simulink model "ExampleVariousBlocks"  (Simulink 9.2)
settings: Solver=FixedStepDiscrete  StartTime=0.0  StopTime=inf  FixedStep=0.001  RelTol=1e-3  EnableMultiTasking=on
InitFcn:
  | RFPRO_TIMESTEP = 1/1000;
  | 
  | % From c-code model
  | gCGHeight = 0.3545;            % height of the car body reference point above the ground
  | gLeftWheelBase = 3.105;        % distance between left front and rear axles
  | gRightWheelBase = 3.105;       % distance between right front and rear axles
  | gFrontTrack = 1.418;           % distance between front left and right wheels
  | gRearTrack = 1.412;            % distance between rear left and right wheels
  | gFrontWheelRadius = 0.32;
  | gRearWheelRadius = 0.33;
  | 
  | CG_OFFSET_FROM_NOSE = [-gLeftWheelBase/2, 0, gCGHeight];
libraries: rFproPhysicsLib x7, simulink x1
settings Model: Creator=enewton  LastModifiedBy=SeanKavanagh  ParamWorkspaceSource=ReferencedWorkspace  TunableVars=LOCAL_PORT_RECV,REMOTE_PORT_RECV,gCGHeight,gFrontTrack,gFrontWheelRadius,gLeftWheelBase,gRearTrack,gRearWheelRadius,gRightWheelBase  TunableVarsStorageClass=Auto,Auto,Auto,Auto,Auto,Auto,Auto,Auto,Auto  TunableVarsTypeQualifier=,,,,,,,,
settings DataIOCC: SaveOutput=off  SignalLogging=off  DSMLogging=off  SaveTime=off
settings OptimizationCC: BlockReduction=off  ConditionallyExecuteInputs=off  OptimizeBlockIOStorage=off  BufferReuse=off  GlobalBufferReuse=off  ExpressionFolding=off  ExpressionDepthLimit=2147483647  LocalBlockOutputs=off  OptimizeDataStoreBuffers=off  BusAssignmentInplaceUpdate=off
settings DebuggingCC: SolverPrmCheckMsg=warning
settings RTWCC: SystemTargetFile=rfpro.tlc  MakeCommand="make_rtw OPTS=\"-DRUN_PHYSICS\""  TemplateMakefile=rfpro.tmf  Description=rFpro Target (Run Physics)  TargetLang=C++
settings STFCustomTargetCC: ModelReferenceCompliant=off  GeneratePreprocessorConditionals=Disable all  CombineOutputUpdateFcns=on  MatFileLogging=on  CPPClassGenCompliant=on  GRTInterface=off  SystemTargetFile=rfpro.tlc
settings GRTTargetCC: ModelReferenceCompliant=off  ParMdlRefBuildCompliant=off  CompOptLevelCompliant=off  ConcurrentExecutionCompliant=off  CombineOutputUpdateFcns=on  GRTInterface=off  UseToolchainInfoCompliant=off

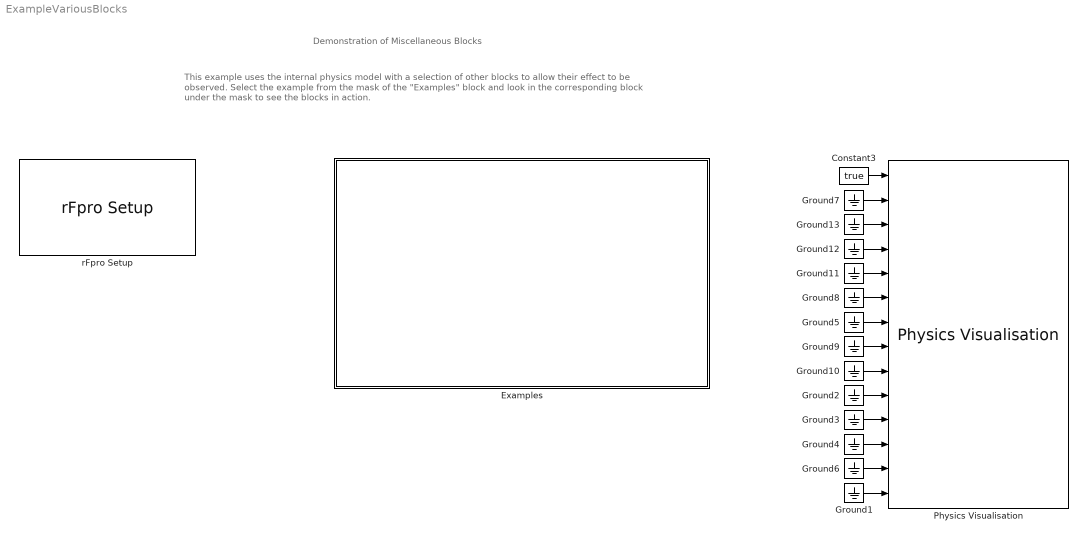
== system ExampleVariousBlocks ==
  note: This example uses the internal physics model with a selection of other blocks to allow their effect to be observed.
      | Select the example from the mask of the "Examples" block and look in the corresponding block under the mask to
      | see the blocks in action.
  note: Demonstration of Miscellaneous Blocks
  Constant3 : Constant  Value=true
  Examples : Subsystem  Variant=on  mask(rFpro Examples){activeExample=Send Command}
      mask prompts: activeExample "Active Example"
      mask help: Select the example you wish to use from the drop down box, and look in the subsystems to see the blocks in use.
      mask init:
      | assignin('base', 'rFpro_VariousBlocksExample', activeExample);
      | 
      | assignin('base', 'rFpro_VariousBlocksCmd', Simulink.Variant('rFpro_VariousBlocksExample == 1'));
      | assignin('base', 'rFpro_VariousBlocksFMOD', Simulink.Variant('rFpro_VariousBlocksExample == 2'));
      | assignin('base', 'rFpro_VariousBlocksTelem', Simulink.Variant('rFpro_VariousBlocksExample == 3'));
      | assignin('base', 'rFpro_VariousBlocksProx', Simulink.Variant('rFpro_VariousBlocksExample == 4'));
      | assignin('base', 'rFpro_VariousBlocksHead', Simulink.Variant('rFpro_VariousBlocksExample == 5'));
      mask TypeOptions activeExample: Send Command | FMOD Sound | Telemetry | Object Proximity | Head Tracking
      mask Display:
      | disp(['Current Example:\n\n' get_param(gcb, 'activeExample')])
      | if activeExample < 4
      |     text(0.2, 0.2, 'Note: external settings required. See under mask.')
      | end
  Ground{1..13} (13 alike) : Ground
  Physics Visualisation : rFproPhysicsLib/Physics Visualisation  PAR_SKIP_INTERNAL_PHYSICS=off  PAR_ACCEL_VALID=off  PAR_ROT_ACCEL_VALID=off  PAR_GEAR_VALID=off  PAR_RPM_VALID=on  PAR_INPUTS_VALID=on  PAR_STEER_TORQUE_VALID=on  PAR_HEADLIGHTS_ON_VALID=off  PAR_WHEEL_POS_VALID=off  PAR_WHEEL_ORI_VALID=off  PAR_TYRE_PARAMS_VALID=off  PAR_WHEEL_ROTATION_VALID=off  PAR_WHEEL_BRAKE_TEMP_VALID=off  PAR_WHEEL_TREAD_TEMP_VALID=off  PAR_WHEEL_AIR_TEMP_VALID=off  period=-1  offset=0  useReverseByteOrder=on  rFpro__platform=Remote Model - Default
  rFpro Setup : rFproPhysicsLib/rFpro Setup  platform=Remote Model - Default  stopOnSessionEnd=on  usePseudoRealtime=on  syncToRF=on  useReverseByteOrder=off  useRfTime=on  minIterations=4  maxIterations=1000  ipReceiveAddress='127.0.0.1'  ipReceivePort=11054  receiveSampleTime=-1  ipTransmitAddress='127.0.0.1'  ipTransmitPort=11052  transmitSampleTime=-1  pluginType=RUN_PHYSICS  sysTarget=xpctarget.tlc  templateMakeFile=xpc_default_tmf  makeCommand=make_rtw  buildDesc=xPC target
  wires:
  Constant3/1 -> Physics Visualisation/1
  Ground13/1 -> Physics Visualisation/3
  Ground12/1 -> Physics Visualisation/4
  Ground11/1 -> Physics Visualisation/5
  Ground8/1 -> Physics Visualisation/6
  Ground5/1 -> Physics Visualisation/7
  Ground9/1 -> Physics Visualisation/8
  Ground10/1 -> Physics Visualisation/9
  Ground2/1 -> Physics Visualisation/10
  Ground3/1 -> Physics Visualisation/11
  Ground4/1 -> Physics Visualisation/12
  Ground6/1 -> Physics Visualisation/13
  Ground1/1 -> Physics Visualisation/14
  Ground7/1 -> Physics Visualisation/2

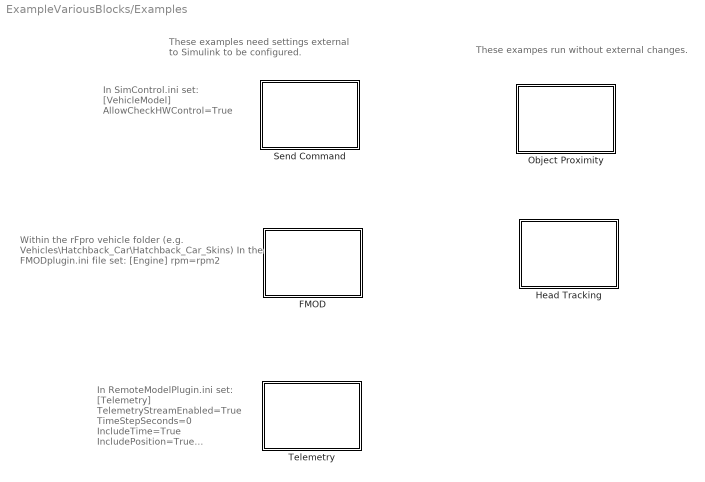
== system ExampleVariousBlocks/Examples ==
  note: These exampes run without external changes.
  note: Within the rFpro vehicle folder
      | (e.g. Vehicles\Hatchback_Car\Hatchback_Car_Skins)
      |
      | In the FMODplugin.ini file set:
      |
      | [Engine]
      | rpm=rpm2
  note: In RemoteModelPlugin.ini set:
      |
      | [Telemetry]
      | TelemetryStreamEnabled=True
      | TimeStepSeconds=0
      | IncludeTime=True
      | IncludePosition=True
      | IncludeDriverControls=True
      | IncludeLapDistance=True
      | IncludeOrientation=True
      | IncludeVelocity=True
      | IncludeRotation=True
      | IncludeLapRef=True
  note: In SimControl.ini set:
      |
      | [VehicleModel]
      | AllowCheckHWControl=True
  note: These examples need settings
      | external to Simulink to be configured.
  FMOD : Subsystem  VariantControl=rFpro_VariousBlocksFMOD
  Head Tracking : Subsystem  VariantControl=rFpro_VariousBlocksHead
  Object Proximity : Subsystem  VariantControl=rFpro_VariousBlocksProx
  Send Command : Subsystem  VariantControl=rFpro_VariousBlocksCmd
  Telemetry : Subsystem  VariantControl=rFpro_VariousBlocksTelem

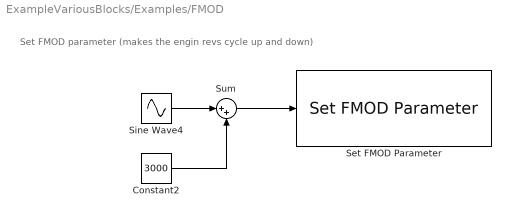
== system ExampleVariousBlocks/Examples/FMOD ==
  note: Set FMOD parameter (makes the engin revs cycle up and down)
  Constant2 : Constant  Value=3000
  Set FMOD Parameter : rFproPhysicsLib/Set FMOD Parameter  parameter_name='rpm2'  useReverseByteOrder=off  rFpro__platform=Remote Model - Default
  Sine Wave4 : Sin  Amplitude=2000  Frequency=2*pi/10
  Sum : Sum  Inputs=|++
  wires:
  Sum/1 -> Set FMOD Parameter/1
  Sine Wave4/1 -> Sum/1
  Constant2/1 -> Sum/2

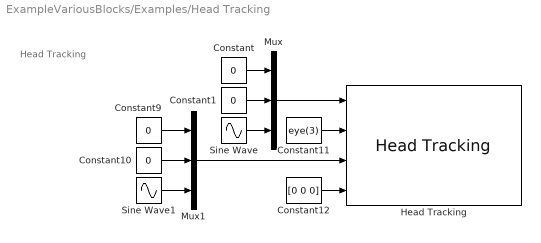
== system ExampleVariousBlocks/Examples/Head Tracking ==
  note: Head Tracking
  Constant{,1,9..10} (4 alike) : Constant  Value=0
  Constant11 : Constant  Value=eye(3)
  Constant12 : Constant  Value=[0 0 0]
  Head Tracking : rFproPhysicsLib/Head Tracking  period=-1  offset=0  useReverseByteOrder=off  rFpro__platform=Remote Model - Default
  Mux : Mux  Inputs=3
  Mux1 : Mux  Inputs=3
  Sine Wave : Sin  Frequency=2*pi / 1  SampleTime=0
  Sine Wave1 : Sin  Amplitude=1 * 2*pi / 1  Frequency=2*pi / 1  Phase=pi/2  SampleTime=0
  wires:
  Constant10/1 -> Mux1/2
  Sine Wave1/1 -> Mux1/3
  Mux1/1 -> Head Tracking/3
  Constant1/1 -> Mux/2
  Sine Wave/1 -> Mux/3
  Constant9/1 -> Mux1/1
  Constant11/1 -> Head Tracking/2
  Constant/1 -> Mux/1
  Constant12/1 -> Head Tracking/4
  Mux/1 -> Head Tracking/1

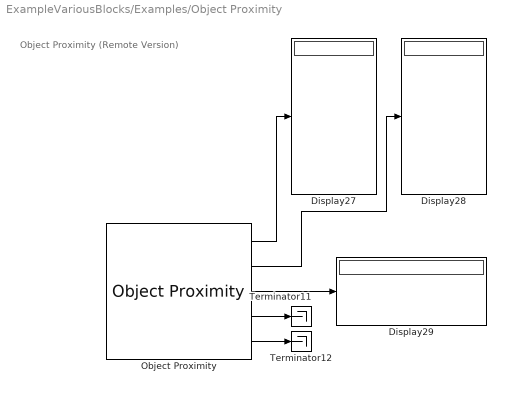
== system ExampleVariousBlocks/Examples/Object Proximity ==
  note: Object Proximity (Remote Version)
  Display27 : Display
  Display28 : Display
  Display29 : Display
  Object Proximity : rFproPhysicsLib/Object Proximity  offsets=[2.0, 0.5, 0.0; 2.0, -0.5, 0.0]'  rays=[0.0, 3.0, 0.0; 0.0, -3.0, 0.0]'  useReverseByteOrder=off  rFpro__platform=Remote Model - Default
  Terminator11 : Terminator
  Terminator12 : Terminator
  wires:
  Object Proximity/2 -> Display28/1
  Object Proximity/4 -> Terminator11/1
  Object Proximity/5 -> Terminator12/1
  Object Proximity/1 -> Display27/1
  Object Proximity/3 -> Display29/1

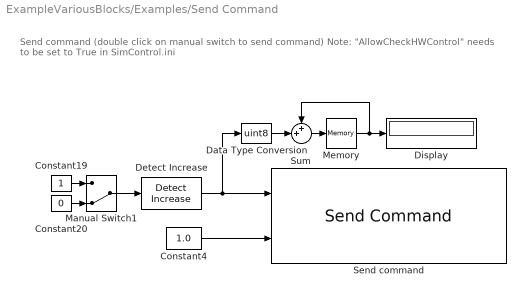
== system ExampleVariousBlocks/Examples/Send Command ==
  note: Send command (double click on manual switch to send command)
      |
      | Note: "AllowCheckHWControl" needs to be set to True in SimControl.ini
  Constant19 : Constant
  Constant20 : Constant  Value=0
  Constant4 : Constant  Value=1.0
  Data Type Conversion : DataTypeConversion  OutDataTypeStr=uint8
  Detect Increase : simulink/Logic and Bit Operations/Detect Increase  vinit=0.0  OutDataTypeStr=boolean
  Display : Display
  Manual Switch1 : ManualSwitch  CurrentSetting=0
  Memory : Memory
  Send command : rFproPhysicsLib/Send Command  presetCmdString=Wipers  customCmdString=CycleOnboard  useCustomStr=off  cmdString=0  useReverseByteOrder=off  rFpro__platform=Remote Model - Default
  Sum : Sum  Inputs=++|
  wires:
  Constant19/1 -> Manual Switch1/1
  Constant20/1 -> Manual Switch1/2
  Manual Switch1/1 -> Detect Increase/1
  Constant4/1 -> Send command/2
  Detect Increase/1 -> Send command/1, Data Type Conversion/1
  Memory/1 -> Sum/1, Display/1
  Sum/1 -> Memory/1
  Data Type Conversion/1 -> Sum/2

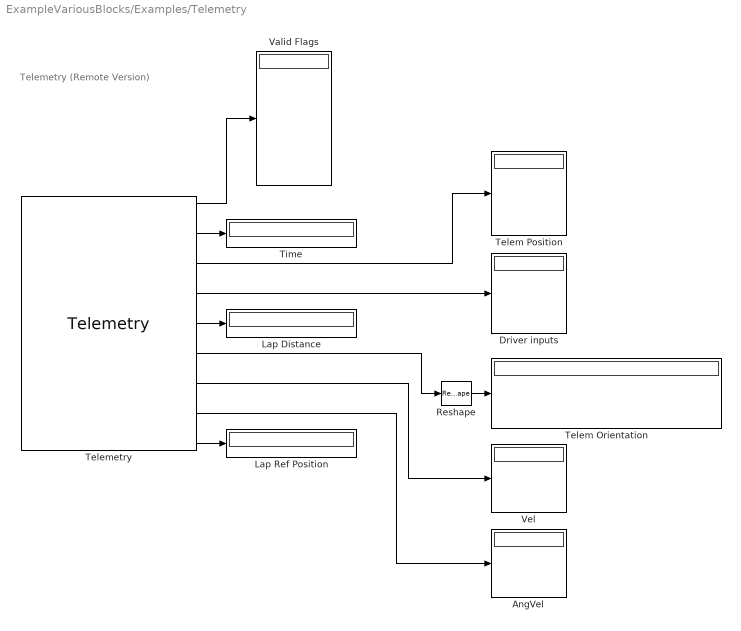
== system ExampleVariousBlocks/Examples/Telemetry ==
  note: Telemetry (Remote Version)
  AngVel : Display
  Driver inputs : Display
  Lap Distance : Display
  Lap Ref Position : Display
  Reshape : Reshape  OutputDimensionality=Customize  OutputDimensions=[3,3]
  Telem Orientation : Display
  Telem Position : Display
  Telemetry : rFproPhysicsLib/Telemetry  pick_Valid=on  pick_Time=on  pick_Pos=on  pick_Driver=on  pick_Lap_Dist=on  pick_Ori=on  pick_Vel=on  pick_Ang_Vel=on  pick_Lap_Dist_Ref=on
  Time : Display
  Valid Flags : Display
  Vel : Display
  wires:
  Telemetry/1 -> Valid Flags/1
  Telemetry/2 -> Time/1
  Telemetry/6 -> Reshape/1
  Telemetry/7 -> Vel/1
  Telemetry/8 -> AngVel/1
  Telemetry/3 -> Telem Position/1
  Reshape/1 -> Telem Orientation/1
  Telemetry/4 -> Driver inputs/1
  Telemetry/5 -> Lap Distance/1
  Telemetry/9 -> Lap Ref Position/1
